simulink model "model"  (R2018b)
settings: Solver=VariableStepAuto  StartTime=0.0  StopTime=T_sim  RelTol=1e-3
values from neighbouring files (symbols this model uses):
  P_elektrolyzer = 4.6    [model_1.m]
  P_fuelcell = 1.2    [model_1.m]
  P_gen_inertia = 3    [model_1.m]
  P_generator = 7    [model_1.m]
  q_per_Watt = 2    [model_1.m]
  t_step = T_dag / 100000    (= 0.00024)    [model_1.m]
  V_stor = 100    [model_1.m]
settings Model: Creator=fabia  LastModifiedBy=fabia

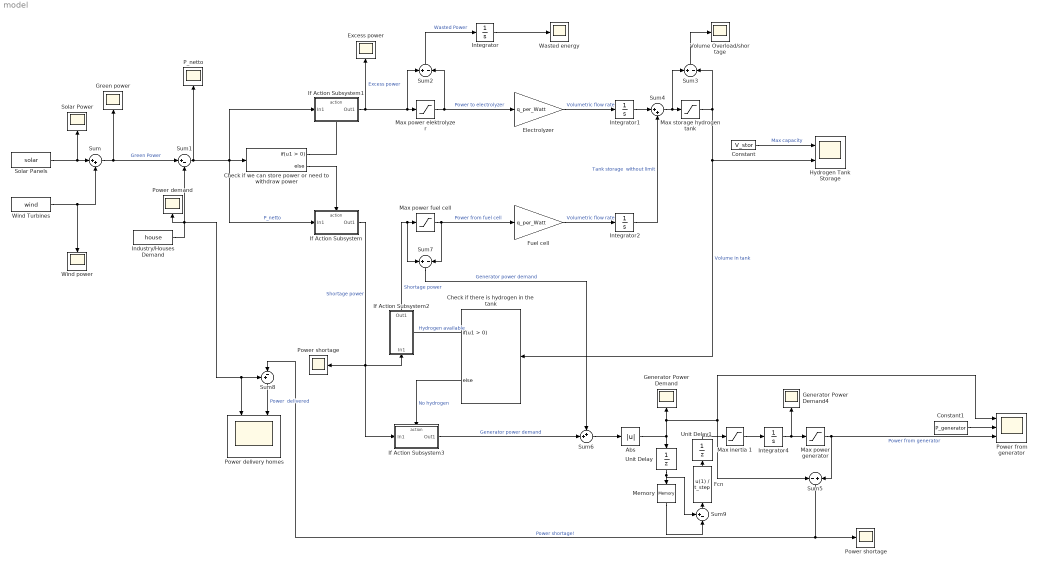
== system model ==
  Abs : Abs
  "Check if there is hydrogen in the tank " : If
  Check if we can store power or need to withdraw power : If
  Constant : Constant  Value=V_stor
  Constant1 : Constant  Value=P_generator
  Electrolyzer : Gain  Gain=q_per_Watt
  Excess power : Scope
  Fcn : Fcn  Expr=u(1) / t_step
  Fuel cell : Gain  Gain=q_per_Watt
  Generator Power Demand : Scope
  Generator Power Demand4 : Scope
  Green power : Scope
  Hydrogen Tank Storage : Scope  NumInputPorts=2
  If Action Subsystem : Subsystem  TreatAsAtomicUnit=on
  If Action Subsystem1 : Subsystem  TreatAsAtomicUnit=on
  If Action Subsystem2 : Subsystem  TreatAsAtomicUnit=on
  If Action Subsystem3 : Subsystem  TreatAsAtomicUnit=on
  Industry/Houses Demand : FromWorkspace  VariableName=house  SampleTime=t_step  Interpolate=off  OutputAfterFinalValue=Setting to zero
  Integrator : Integrator
  Integrator1 : Integrator
  Integrator2 : Integrator
  Integrator4 : Integrator  InitialCondition=0.5
  Max inertia 1 : Saturate  UpperLimit=P_gen_inertia  LowerLimit=-1 * P_gen_inertia
  Max power elektrolyzer : Saturate  UpperLimit=P_elektrolyzer  LowerLimit=0
  Max power fuel cell : Saturate  UpperLimit=0  LowerLimit=-1 * P_fuelcell
  Max power generator : Saturate  UpperLimit=P_generator  LowerLimit=0
  Max storage hydrogen tank : Saturate  UpperLimit=V_stor  LowerLimit=0
  Memory : Memory  InitialCondition=0.5
  P_netto : Scope
  Power delivery homes : Scope  NumInputPorts=2
  Power demand : Scope
  Power from generator : Scope  NumInputPorts=3
  Power shortage : Scope
  "Power shortage " : Scope
  Solar Panels : FromWorkspace  VariableName=solar  SampleTime=t_step  Interpolate=off  OutputAfterFinalValue=Setting to zero
  Solar Power : Scope
  Sum : Sum  Inputs=|++
  Sum1 : Sum  Inputs=|+-
  Sum2 : Sum  Inputs=+-
  Sum3 : Sum  Inputs=+-
  Sum4 : Sum  Inputs=|++
  Sum5 : Sum  Inputs=-+
  Sum6 : Sum  Inputs=++|
  Sum7 : Sum  Inputs=+-
  Sum8 : Sum  Inputs=+-|
  Sum9 : Sum  Inputs=+-|
  Unit Delay : UnitDelay  InitialCondition=0.5  SampleTime=t_step
  Unit Delay1 : UnitDelay  SampleTime=t_step
  Volume Overload/shortage : Scope
  Wasted energy : Scope
  Wind Turbines : FromWorkspace  VariableName=wind  SampleTime=t_step  Interpolate=off  OutputAfterFinalValue=Setting to zero
  Wind power : Scope
  wires:
  Sum/1 -> Green power/1, Sum1/1  "Green Power"
  Sum1/1 -> P_netto/1, If Action Subsystem1/1(In1), If Action Subsystem/1(In1), Check if we can store power or need to withdraw power/1  "P_netto"
  Check if we can store power or need to withdraw power/2 -> If Action Subsystem/Action
  Check if we can store power or need to withdraw power/1 -> If Action Subsystem1/Action
  If Action Subsystem1/1(Out1) -> Sum2/1, Max power elektrolyzer/1, Excess power/1  "Excess power"
  Max power elektrolyzer/1 -> Sum2/2, Electrolyzer/1  "Power to electrolyzer"
  Sum2/1 -> Integrator/1  "Wasted Power"
  Integrator/1 -> Wasted energy/1
  Electrolyzer/1 -> Integrator1/1  "Volumetric flow rate"
  Constant/1 -> Hydrogen Tank Storage/1  "Max capacity"
  Integrator1/1 -> Sum4/1
  Sum3/1 -> Volume Overload/shortage/1
  Max storage hydrogen tank/1 -> "Check if there is hydrogen in the tank "/1, Hydrogen Tank Storage/2, Sum3/2  "Volume in tank"
  If Action Subsystem/1(Out1) -> Power shortage/1, If Action Subsystem3/1(In1), If Action Subsystem2/1(In1)  "Shortage power"
  Max power fuel cell/1 -> Sum7/2, Fuel cell/1  "Power from fuel cell"
  Fuel cell/1 -> Integrator2/1  "Volumetric flow rate"
  Sum4/1 -> Sum3/1, Max storage hydrogen tank/1
  Integrator2/1 -> Sum4/2  "Tank storage  without limit"
  "Check if there is hydrogen in the tank "/1 -> If Action Subsystem2/Action  "Hydrogen available"
  "Check if there is hydrogen in the tank "/2 -> If Action Subsystem3/Action  "No hydrogen"
  If Action Subsystem2/1(Out1) -> Sum7/1, Max power fuel cell/1  "Shortage power"
  Max power generator/1 -> Power from generator/3, Sum5/2  "Power from generator"
  If Action Subsystem3/1(Out1) -> Sum6/2  "Generator power demand"
  Sum7/1 -> Sum6/1  "Generator power demand"
  Sum8/1 -> Power delivery homes/2  "Power  delivered"
  Solar Panels/1 -> Solar Power/1, Sum/1
  Constant1/1 -> Power from generator/2
  Industry/Houses Demand/1 -> Power delivery homes/1, Sum8/1, Sum1/2, Power demand/1
  Wind Turbines/1 -> Sum/2, Wind power/1
  Sum6/1 -> Abs/1
  Abs/1 -> Power from generator/1, Sum5/1, Generator Power Demand/1, Unit Delay/1
  Sum5/1 -> Sum8/2, "Power shortage "/1  "Power shortage!"
  Unit Delay/1 -> Sum9/1, Memory/1
  Fcn/1 -> Unit Delay1/1
  Sum9/1 -> Fcn/1
  Memory/1 -> Sum9/2
  Unit Delay1/1 -> Max inertia 1/1
  Max inertia 1/1 -> Integrator4/1
  Integrator4/1 -> Max power generator/1, Generator Power Demand4/1

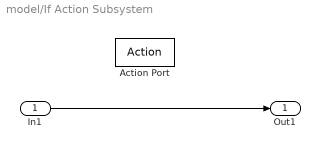
== system model/If Action Subsystem ==
  In1 : Inport
  Action Port : ActionPort  ActionType=else
  Out1 : Outport
  wires:
  In1/1 -> Out1/1

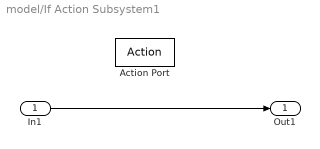
== system model/If Action Subsystem1 ==
  In1 : Inport
  Action Port : ActionPort  ActionType=then
  Out1 : Outport
  wires:
  In1/1 -> Out1/1

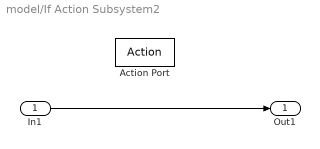
== system model/If Action Subsystem2 ==
  In1 : Inport
  Action Port : ActionPort  ActionType=then
  Out1 : Outport
  wires:
  In1/1 -> Out1/1

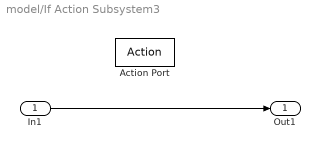
== system model/If Action Subsystem3 ==
  In1 : Inport
  Action Port : ActionPort  ActionType=else
  Out1 : Outport
  wires:
  In1/1 -> Out1/1
